simulink model "SYNC"  (R2019b)
settings: Solver=FixedStepAuto  StartTime=0.0  StopTime=10  FixedStep=0.1  RelTol=1e-3
settings Model: Creator=JDALUZ1  LastModifiedBy=EMORAI12
settings SolverCC: PositivePriorityOrder=on  AutoInsertRateTranBlk=on  InsertRTBMode=Always
settings DebuggingCC: ArithmeticOperatorsInVariantConditions=warning
settings SFSimCC: CustomCodeUndefinedFunction=UseInterfaceOnly
settings CodeAppCC: StateflowObjectComments=on

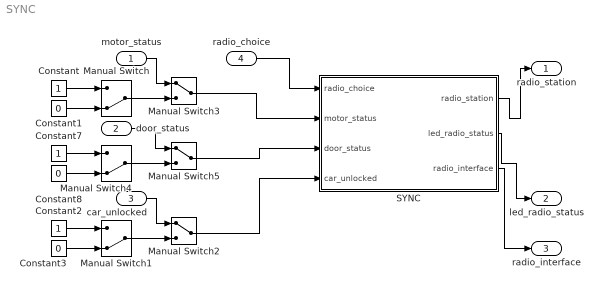
== system SYNC ==
  motor_status : Inport
  door_status : Inport  Port=2
  car_unlocked : Inport  Port=3
  radio_choice : Inport  Port=4
  Constant : Constant
  Constant1 : Constant  Value=0
  Constant2 : Constant
  Constant3 : Constant  Value=0
  Constant7 : Constant
  Constant8 : Constant  Value=0
  Manual Switch : ManualSwitch  CurrentSetting=0
  Manual Switch1 : ManualSwitch  CurrentSetting=0
  Manual Switch2 : ManualSwitch
  Manual Switch3 : ManualSwitch
  Manual Switch4 : ManualSwitch  CurrentSetting=0
  Manual Switch5 : ManualSwitch
  SYNC : Stateflow chart  TreatAsAtomicUnit=on
  radio_station : Outport
  led_radio_status : Outport  Port=2
  radio_interface : Outport  Port=3
  wires:
  SYNC/1(radio_station) -> radio_station/1
  SYNC/2(led_radio_status) -> led_radio_status/1
  Constant/1 -> Manual Switch/1
  Constant1/1 -> Manual Switch/2
  Manual Switch/1 -> Manual Switch3/2
  motor_status/1 -> Manual Switch3/1
  Manual Switch3/1 -> SYNC/2(motor_status)
  Manual Switch4/1 -> Manual Switch5/2
  door_status/1 -> Manual Switch5/1
  Manual Switch5/1 -> SYNC/3(door_status)
  Constant8/1 -> Manual Switch4/2
  Constant7/1 -> Manual Switch4/1
  Manual Switch1/1 -> Manual Switch2/2
  car_unlocked/1 -> Manual Switch2/1
  Manual Switch2/1 -> SYNC/4(car_unlocked)
  Constant3/1 -> Manual Switch1/2
  Constant2/1 -> Manual Switch1/1
  SYNC/3(radio_interface) -> radio_interface/1
  radio_choice/1 -> SYNC/1(radio_choice)

== stateflow chart SYNC/SYNC ==
  state radio_switching
    note: Do not put any code along
        | the transitions that run
        | down the right side!
    (default) -> (junction 124) : %radio switching
    (junction 124) -> (junction 125) [order 1] : [radio_choice == Bahia_FM]
    (junction 124) -> (junction 128) [order 2]
    (junction 125) -> (junction 126) : {radio_station=88.7;}
    (junction 126) -> (junction 127)
    (junction 127) -> (junction 131)
    (junction 128) -> (junction 129) [order 1] : [radio_choice == Globo_FM]
    (junction 128) -> (junction 132) [order 2]
    (junction 129) -> (junction 130) : {radio_station=90.1;}
    (junction 130) -> (junction 131)
    (junction 131) -> (junction 135)
    (junction 132) -> (junction 133) [order 1] : [radio_choice == Jovenpan]
    (junction 132) -> (junction 136) [order 2]
    (junction 133) -> (junction 134) : {radio_station=91.3;}
    (junction 134) -> (junction 135)
    (junction 135) -> (junction 139)
    (junction 136) -> (junction 137) [order 1] : [radio_choice == transamericapop]
    (junction 136) -> (junction 140) [order 2] : {radio_station=88.7;}
    (junction 137) -> (junction 138) : {radio_station=100.1;}
    (junction 138) -> (junction 139)
    (junction 139) -> (junction 141)
    (junction 141) -> (junction 140)
    (junction 140) -> (junction 142)
  state door_unlock_and_open
    entry:
    lock_unlock=1;%porta destrancada
    during:
    if (door_status==1)%se porta entreaberta
    radio_interface=1; %interface de radio wellcome
    led_radio_status=1; %led indicador on
    elseif (door_status==0)%se porta fechada
    radio_interface=0;%interface de radio off
    led_radio_status=0;%led indicador off
    end
  note: %verificando se a porta foi destravada
  note: %verifica se há porta entreaberta
  state wellcome_and_radio_interface
    entry:
    %if (radio_interface==1)
    radio_station=0;
    %after (5 , sec):
    %end
    exit:
    radio_interface=2;
  state door_lock_and_closed
    entry:
    radio_station=1; %blackout radio
    radio_interface=0; %interface de radio off
    led_radio_status=0;%led indicador off
    lock_unlock=0;%porta trancada
  (default) -> door_lock_and_closed
  door_lock_and_closed -> door_unlock_and_open : [car_unlocked==1 ]
  radio_switching -> radio_switching [order 2] : after(500,msec)
  door_unlock_and_open -> wellcome_and_radio_interface [order 1] : [ door_status==1 && led_radio_status==1]
  door_unlock_and_open -> door_lock_and_closed [order 2] : [car_unlocked==0 ]
  wellcome_and_radio_interface -> radio_switching : after(5,sec)
  (junction 155) -> door_lock_and_closed
  radio_switching -> (junction 155) [order 1] : [car_unlocked==0 ]
  data: radio_station output; Bahia_FM constant double =88.7; Globo_FM constant double =90.1; radio_choice input; transamericapop constant double =100.1; Jovenpan constant double =91.3; led_radio_status output; lock_unlock local; motor_status input; door_status input; car_unlocked input; radio_interface output
